simulink model "pid_4"  (Simulink 6.0)
settings: Solver=ode45  StartTime=0.0  StopTime=30  RelTol=1e-3
undefined symbols (not defined in the file): DiscIntNeverNeededParam
libraries: simulink x1
settings Model: LastModifiedBy=star

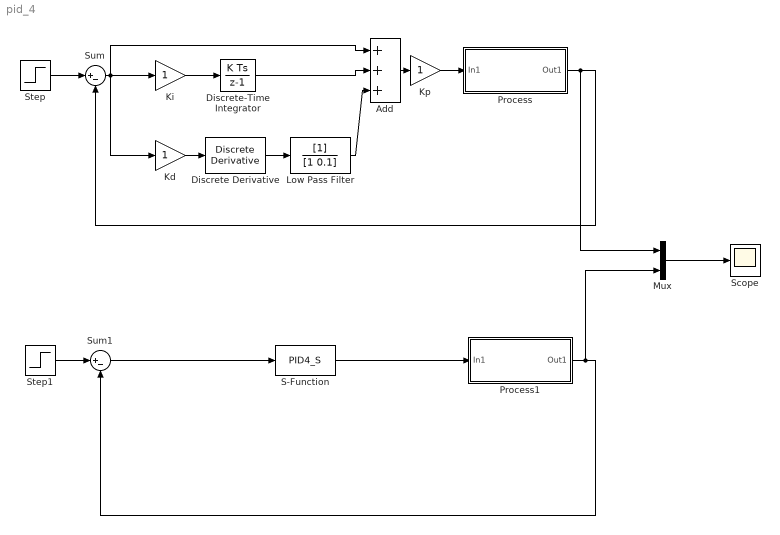
== system pid_4 ==
  Add : Sum  Inputs=+++  OutScaling=2^-10
  Discrete Derivative : simulink/Discrete/Discrete Derivative  gainval=1.0  ICPrevScaledInput=0.0  OutDataType=sfix(16)  OutScaling=2^-10  DoSatur=off
  Discrete-Time Integrator : DiscreteIntegrator  ICPrevOutput=DiscIntNeverNeededParam  ICPrevScaledInput=DiscIntNeverNeededParam
  Kd : Gain  SampleTime=1
  Ki : Gain  SampleTime=1
  Kp : Gain  SampleTime=1
  Low Pass Filter : DiscreteFilter  Denominator=[1 0.1]
  Mux : Mux  Inputs=2
  Process : Subsystem
  Process1 : Subsystem
  S-Function : S-Function  FunctionName=PID4_S  Parameters=1,1,1,1,0.1
  Scope : Scope
  Step : Step  Time=0  SampleTime=0
  Step1 : Step  Time=0  SampleTime=0
  Sum : Sum  Inputs=|+-
  Sum1 : Sum  Inputs=|+-
  wires:
  Sum/1 -> Kd/1, Ki/1, Add/1
  Discrete-Time Integrator/1 -> Add/2
  Ki/1 -> Discrete-Time Integrator/1
  Process/1(Out1) -> Sum/2, Mux/1
  Kd/1 -> Discrete Derivative/1
  Step/1 -> Sum/1
  Add/1 -> Kp/1
  Kp/1 -> Process/1(In1)
  Discrete Derivative/1 -> Low Pass Filter/1
  Low Pass Filter/1 -> Add/3
  Process1/1(Out1) -> Sum1/2, Mux/2
  Step1/1 -> Sum1/1
  S-Function/1 -> Process1/1(In1)
  Sum1/1 -> S-Function/1
  Mux/1 -> Scope/1

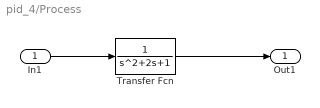
== system pid_4/Process ==
  In1 : Inport  Port=1  LatchInput=off
  Transfer Fcn : TransferFcn
  Out1 : Outport
  wires:
  In1/1 -> Transfer Fcn/1
  Transfer Fcn/1 -> Out1/1

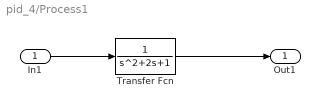
== system pid_4/Process1 ==
  In1 : Inport  Port=1  LatchInput=off
  Transfer Fcn : TransferFcn
  Out1 : Outport
  wires:
  In1/1 -> Transfer Fcn/1
  Transfer Fcn/1 -> Out1/1
